simulink model "scenario_2_TAC_5robots_plus_2019"  (R2020a)
settings: Solver=FixedStepAuto  StartTime=0.0  StopTime=60.0  FixedStep=1e-2  RelTol=1e-3
libraries: simulink x5
(part 1 of 2)
settings Model: Creator=Admin  LastModifiedBy=Admin

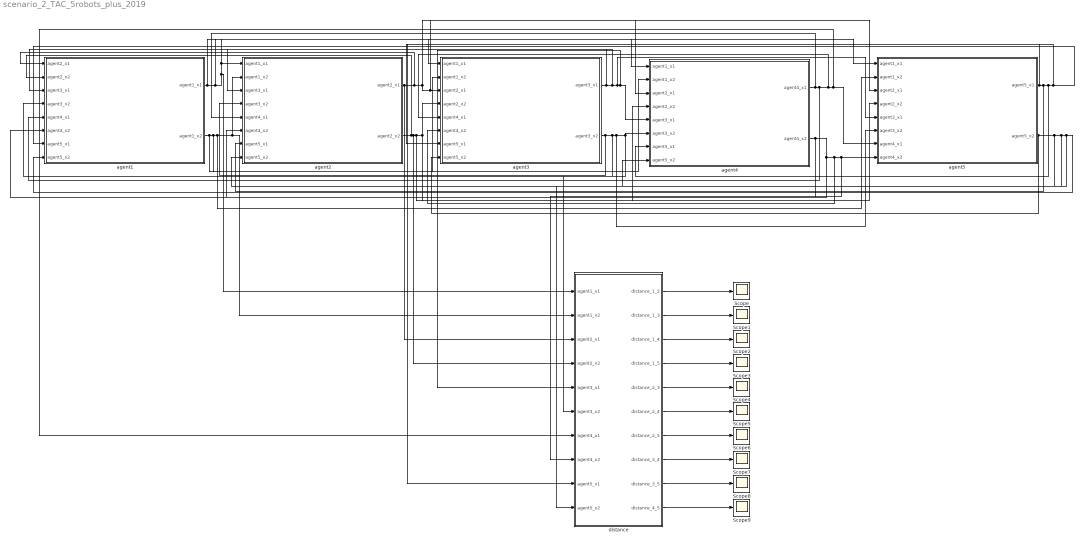
== system scenario_2_TAC_5robots_plus_2019 ==
  Scope{,1..9} (10 alike) : Scope
  agent1 : Subsystem
  agent2 : Subsystem
  agent3 : Subsystem
  agent4 : Subsystem
  agent5 : Subsystem
  distance : MATLAB Function  TreatAsAtomicUnit=on
  wires:
  agent1/1(agent1_x1) -> agent4/1(agent1_x1), agent3/1(agent1_x1), distance/1(agent1_x1), agent5/1(agent1_x1), agent2/1(agent1_x1)
  agent1/2(agent1_x2) -> agent3/2(agent1_x2), agent4/2(agent1_x2), agent5/2(agent1_x2), distance/2(agent1_x2), agent2/2(agent1_x2)
  agent2/1(agent2_x1) -> distance/3(agent2_x1), agent1/1(agent2_x1), agent4/3(agent2_x1), agent3/3(agent2_x1), agent5/3(agent2_x1)
  agent2/2(agent2_x2) -> agent1/2(agent2_x2), distance/4(agent2_x2), agent4/4(agent2_x2), agent5/4(agent2_x2), agent3/4(agent2_x2)
  agent3/1(agent3_x1) -> agent1/3(agent3_x1), agent2/3(agent3_x1), agent5/5(agent3_x1), distance/5(agent3_x1), agent4/5(agent3_x1)
  agent3/2(agent3_x2) -> agent2/4(agent3_x2), agent1/4(agent3_x2), agent5/6(agent3_x2), distance/6(agent3_x2), agent4/6(agent3_x2)
  agent4/1(agent4_x1) -> agent2/5(agent4_x1), agent1/5(agent4_x1), agent3/5(agent4_x1), distance/7(agent4_x1), agent5/7(agent4_x1)
  agent4/2(agent4_x2) -> agent1/6(agent4_x2), agent2/6(agent4_x2), agent3/6(agent4_x2), distance/8(agent4_x2), agent5/8(agent4_x2)
  agent5/1(agent5_x1) -> agent3/7(agent5_x1), agent2/7(agent5_x1), agent4/7(agent5_x1), distance/9(agent5_x1), agent1/7(agent5_x1)
  agent5/2(agent5_x2) -> agent4/8(agent5_x2), distance/10(agent5_x2), agent1/8(agent5_x2), agent2/8(agent5_x2), agent3/8(agent5_x2)
  distance/1(distance_1_2) -> Scope/1
  distance/2(distance_1_3) -> Scope1/1
  distance/3(distance_1_4) -> Scope2/1
  distance/4(distance_1_5) -> Scope3/1
  distance/5(distance_2_3) -> Scope4/1
  distance/6(distance_2_4) -> Scope5/1
  distance/7(distance_2_5) -> Scope6/1
  distance/8(distance_3_4) -> Scope7/1
  distance/9(distance_3_5) -> Scope8/1
  distance/10(distance_4_5) -> Scope9/1

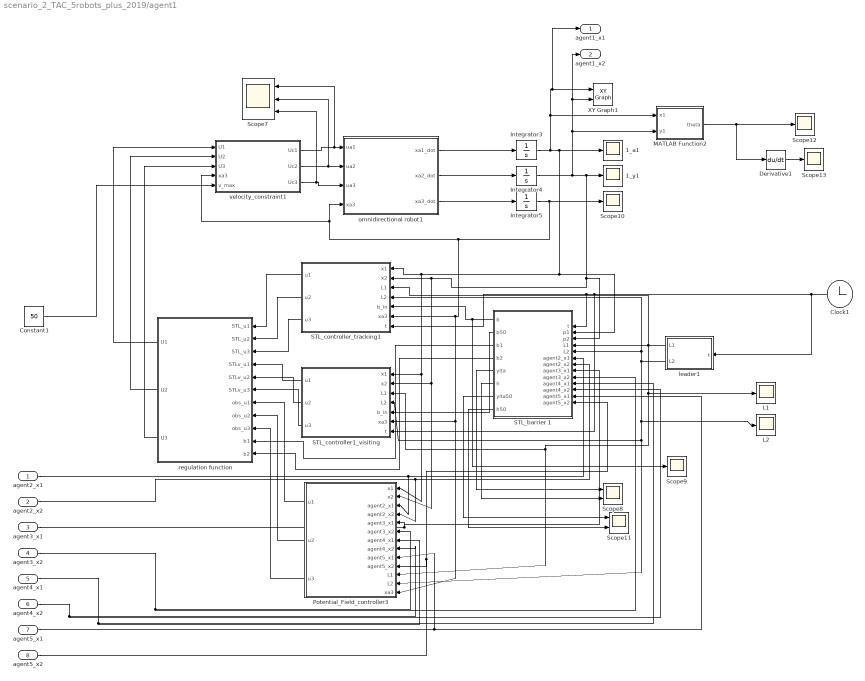
== system scenario_2_TAC_5robots_plus_2019/agent1 ==
  agent2_x1 : Inport
  agent2_x2 : Inport  Port=2
  agent3_x1 : Inport  Port=3
  agent3_x2 : Inport  Port=4
  agent4_x1 : Inport  Port=5
  agent4_x2 : Inport  Port=6
  agent5_x1 : Inport  Port=7
  agent5_x2 : Inport  Port=8
  1_a1 : Scope
  1_y1 : Scope
  Clock1 : Clock
  Constant1 : Constant  Value=50
  Derivative1 : Derivative
  Integrator3 : Integrator
  Integrator4 : Integrator  InitialCondition=10
  Integrator5 : Integrator
  L1 : Scope
  L2 : Scope
  MATLAB Function2 : MATLAB Function  TreatAsAtomicUnit=on
  Potential_Field_controller3 : MATLAB Function  TreatAsAtomicUnit=on
  STL_barrier 1 : MATLAB Function  TreatAsAtomicUnit=on
  STL_controller1_visiting : MATLAB Function  TreatAsAtomicUnit=on
  STL_controller_tracking1 : MATLAB Function  TreatAsAtomicUnit=on
  Scope{9..10,12..13} (4 alike) : Scope
  Scope11 : Scope  NumInputPorts=2
  Scope7 : Scope  NumInputPorts=3
  Scope8 : Scope  NumInputPorts=2
  XY Graph1 : simulink/Sinks/XY Graph  xmin=-60  xmax=60  ymin=-60  ymax=60  st=0.01
  leader1 : MATLAB Function  TreatAsAtomicUnit=on
  omnidirectional robot1 : MATLAB Function  TreatAsAtomicUnit=on
  "regulation function " : MATLAB Function  TreatAsAtomicUnit=on
  velocity_constraint1 : MATLAB Function  TreatAsAtomicUnit=on
  agent1_x1 : Outport
  agent1_x2 : Outport  Port=2
  wires:
  velocity_constraint1/1(Uc1) -> Scope7/1, omnidirectional robot1/1(ua1)
  Integrator3/1 -> MATLAB Function2/1(x1), agent1_x1/1, XY Graph1/1, STL_barrier 1/2(p1), Potential_Field_controller3/1(x1), STL_controller1_visiting/1(x1), STL_controller_tracking1/1(x1), 1_a1/1
  Potential_Field_controller3/3(u3) -> "regulation function "/9(obs_u3)
  omnidirectional robot1/1(xa1_dot) -> Integrator3/1
  leader1/2(L2) -> STL_barrier 1/5(L2), STL_controller_tracking1/4(L2), STL_controller1_visiting/4(L2), Potential_Field_controller3/12(L2), L2/1
  Constant1/1 -> velocity_constraint1/5(v_max)
  STL_barrier 1/4(b2) -> "regulation function "/11(b2)
  Clock1/1 -> STL_controller_tracking1/7(t), STL_barrier 1/1(t), STL_controller1_visiting/7(t), leader1/1(t)
  MATLAB Function2/1(theta) -> Derivative1/1, Scope12/1
  "regulation function "/3(U3) -> velocity_constraint1/3(U3)
  Integrator4/1 -> MATLAB Function2/2(y1), agent1_x2/1, XY Graph1/2, Potential_Field_controller3/2(x2), STL_controller1_visiting/2(x2), STL_controller_tracking1/2(x2), STL_barrier 1/3(p2), 1_y1/1
  omnidirectional robot1/3(xa3_dot) -> Integrator5/1
  STL_controller_tracking1/2(u2) -> "regulation function "/2(STL_u2)
  Potential_Field_controller3/2(u2) -> "regulation function "/8(obs_u2)
  STL_barrier 1/5(yita) -> Scope8/1
  omnidirectional robot1/2(xa2_dot) -> Integrator4/1
  velocity_constraint1/2(Uc2) -> Scope7/2, omnidirectional robot1/2(ua2)
  Potential_Field_controller3/1(u1) -> "regulation function "/7(obs_u1)
  STL_controller_tracking1/3(u3) -> "regulation function "/3(STL_u3)
  STL_barrier 1/6(h) -> Scope8/2
  STL_barrier 1/1(b) -> STL_controller_tracking1/5(b_in), Scope9/1
  STL_barrier 1/3(b1) -> "regulation function "/10(b1)
  STL_barrier 1/8(h50) -> Scope11/2
  velocity_constraint1/3(Uc3) -> Scope7/3, omnidirectional robot1/3(ua3)
  STL_barrier 1/2(b50) -> STL_controller1_visiting/5(b_in)
  "regulation function "/1(U1) -> velocity_constraint1/1(U1)
  leader1/1(L1) -> L1/1, Potential_Field_controller3/11(L1), STL_controller1_visiting/3(L1), STL_barrier 1/4(L1), STL_controller_tracking1/3(L1)
  Integrator5/1 -> velocity_constraint1/4(xa3), omnidirectional robot1/4(xa3), Potential_Field_controller3/13(xa3), STL_controller1_visiting/6(xa3), STL_controller_tracking1/6(xa3), Scope10/1
  Derivative1/1 -> Scope13/1
  STL_barrier 1/7(yita50) -> Scope11/1
  STL_controller1_visiting/3(u3) -> "regulation function "/6(STLv_u3)
  "regulation function "/2(U2) -> velocity_constraint1/2(U2)
  STL_controller1_visiting/1(u1) -> "regulation function "/4(STLv_u1)
  STL_controller1_visiting/2(u2) -> "regulation function "/5(STLv_u2)
  STL_controller_tracking1/1(u1) -> "regulation function "/1(STL_u1)
  agent2_x1/1 -> STL_barrier 1/6(agent2_x1), Potential_Field_controller3/3(agent2_x1)
  agent2_x2/1 -> STL_barrier 1/7(agent2_x2), Potential_Field_controller3/4(agent2_x2)
  agent3_x1/1 -> STL_barrier 1/8(agent3_x1), Potential_Field_controller3/5(agent3_x1)
  agent3_x2/1 -> STL_barrier 1/9(agent3_x2), Potential_Field_controller3/6(agent3_x2)
  agent4_x1/1 -> STL_barrier 1/10(agent4_x1), Potential_Field_controller3/7(agent4_x1)
  agent4_x2/1 -> STL_barrier 1/11(agent4_x2), Potential_Field_controller3/8(agent4_x2)
  agent5_x1/1 -> STL_barrier 1/12(agent5_x1), Potential_Field_controller3/9(agent5_x1)
  agent5_x2/1 -> STL_barrier 1/13(agent5_x2), Potential_Field_controller3/10(agent5_x2)

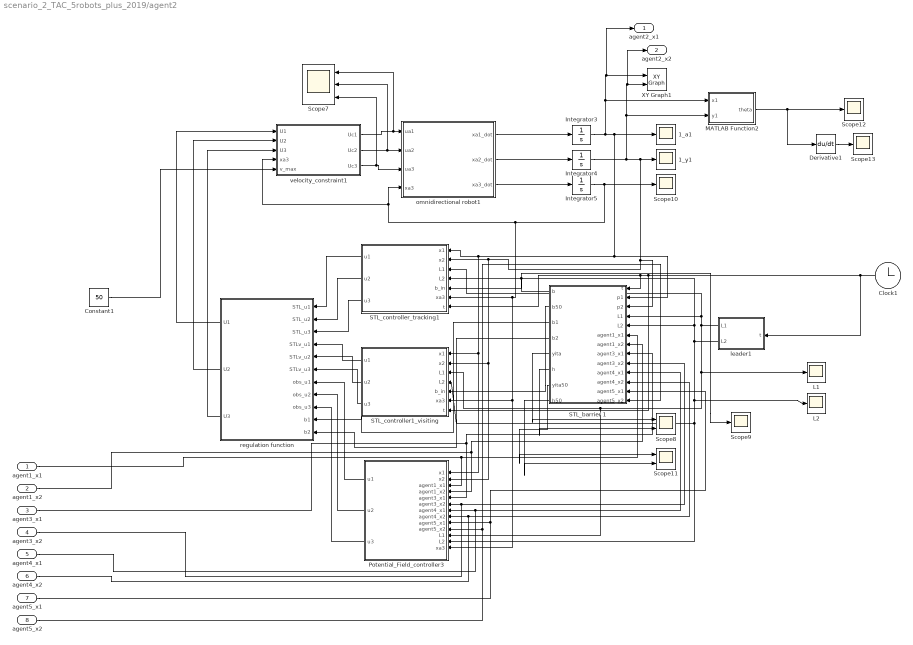
== system scenario_2_TAC_5robots_plus_2019/agent2 ==
  agent1_x1 : Inport
  agent1_x2 : Inport  Port=2
  agent3_x1 : Inport  Port=3
  agent3_x2 : Inport  Port=4
  agent4_x1 : Inport  Port=5
  agent4_x2 : Inport  Port=6
  agent5_x1 : Inport  Port=7
  agent5_x2 : Inport  Port=8
  1_a1 : Scope
  1_y1 : Scope
  Clock1 : Clock
  Constant1 : Constant  Value=50
  Derivative1 : Derivative
  Integrator3 : Integrator  InitialCondition=10
  Integrator4 : Integrator
  Integrator5 : Integrator
  L1 : Scope
  L2 : Scope
  MATLAB Function2 : MATLAB Function  TreatAsAtomicUnit=on
  Potential_Field_controller3 : MATLAB Function  TreatAsAtomicUnit=on
  STL_barrier 1 : MATLAB Function  TreatAsAtomicUnit=on
  STL_controller1_visiting : MATLAB Function  TreatAsAtomicUnit=on
  STL_controller_tracking1 : MATLAB Function  TreatAsAtomicUnit=on
  Scope{9..10,12..13} (4 alike) : Scope
  Scope11 : Scope  NumInputPorts=2
  Scope7 : Scope  NumInputPorts=3
  Scope8 : Scope  NumInputPorts=2
  XY Graph1 : simulink/Sinks/XY Graph  xmin=-60  xmax=60  ymin=-60  ymax=60  st=0.01
  leader1 : MATLAB Function  TreatAsAtomicUnit=on
  omnidirectional robot1 : MATLAB Function  TreatAsAtomicUnit=on
  "regulation function " : MATLAB Function  TreatAsAtomicUnit=on
  velocity_constraint1 : MATLAB Function  TreatAsAtomicUnit=on
  agent2_x1 : Outport
  agent2_x2 : Outport  Port=2
  wires:
  velocity_constraint1/1(Uc1) -> Scope7/1, omnidirectional robot1/1(ua1)
  Integrator3/1 -> MATLAB Function2/1(x1), agent2_x1/1, XY Graph1/1, STL_barrier 1/2(p1), Potential_Field_controller3/1(x1), STL_controller1_visiting/1(x1), STL_controller_tracking1/1(x1), 1_a1/1
  Potential_Field_controller3/3(u3) -> "regulation function "/9(obs_u3)
  omnidirectional robot1/1(xa1_dot) -> Integrator3/1
  leader1/2(L2) -> STL_controller_tracking1/4(L2), STL_barrier 1/5(L2), STL_controller1_visiting/4(L2), Potential_Field_controller3/12(L2), L2/1
  Constant1/1 -> velocity_constraint1/5(v_max)
  STL_barrier 1/4(b2) -> "regulation function "/11(b2)
  Clock1/1 -> STL_controller_tracking1/7(t), STL_barrier 1/1(t), STL_controller1_visiting/7(t), leader1/1(t)
  MATLAB Function2/1(theta) -> Derivative1/1, Scope12/1
  "regulation function "/3(U3) -> velocity_constraint1/3(U3)
  Integrator4/1 -> MATLAB Function2/2(y1), agent2_x2/1, XY Graph1/2, Potential_Field_controller3/2(x2), STL_controller1_visiting/2(x2), STL_controller_tracking1/2(x2), STL_barrier 1/3(p2), 1_y1/1
  omnidirectional robot1/3(xa3_dot) -> Integrator5/1
  STL_controller_tracking1/2(u2) -> "regulation function "/2(STL_u2)
  Potential_Field_controller3/2(u2) -> "regulation function "/8(obs_u2)
  STL_barrier 1/5(yita) -> Scope8/1
  omnidirectional robot1/2(xa2_dot) -> Integrator4/1
  velocity_constraint1/2(Uc2) -> Scope7/2, omnidirectional robot1/2(ua2)
  Potential_Field_controller3/1(u1) -> "regulation function "/7(obs_u1)
  STL_controller_tracking1/3(u3) -> "regulation function "/3(STL_u3)
  STL_barrier 1/6(h) -> Scope8/2
  STL_barrier 1/1(b) -> STL_controller_tracking1/5(b_in), Scope9/1
  STL_barrier 1/3(b1) -> "regulation function "/10(b1)
  STL_barrier 1/8(h50) -> Scope11/2
  velocity_constraint1/3(Uc3) -> Scope7/3, omnidirectional robot1/3(ua3)
  STL_barrier 1/2(b50) -> STL_controller1_visiting/5(b_in)
  "regulation function "/1(U1) -> velocity_constraint1/1(U1)
  leader1/1(L1) -> STL_controller_tracking1/3(L1), STL_barrier 1/4(L1), L1/1, STL_controller1_visiting/3(L1), Potential_Field_controller3/11(L1)
  Integrator5/1 -> velocity_constraint1/4(xa3), omnidirectional robot1/4(xa3), Potential_Field_controller3/13(xa3), STL_controller1_visiting/6(xa3), STL_controller_tracking1/6(xa3), Scope10/1
  Derivative1/1 -> Scope13/1
  STL_barrier 1/7(yita50) -> Scope11/1
  STL_controller1_visiting/3(u3) -> "regulation function "/6(STLv_u3)
  "regulation function "/2(U2) -> velocity_constraint1/2(U2)
  STL_controller1_visiting/1(u1) -> "regulation function "/4(STLv_u1)
  STL_controller1_visiting/2(u2) -> "regulation function "/5(STLv_u2)
  STL_controller_tracking1/1(u1) -> "regulation function "/1(STL_u1)
  agent1_x1/1 -> STL_barrier 1/6(agent1_x1), Potential_Field_controller3/3(agent1_x1)
  agent1_x2/1 -> STL_barrier 1/7(agent1_x2), Potential_Field_controller3/4(agent1_x2)
  agent3_x1/1 -> STL_barrier 1/8(agent3_x1), Potential_Field_controller3/5(agent3_x1)
  agent3_x2/1 -> STL_barrier 1/9(agent3_x2), Potential_Field_controller3/6(agent3_x2)
  agent4_x1/1 -> STL_barrier 1/10(agent4_x1), Potential_Field_controller3/7(agent4_x1)
  agent4_x2/1 -> STL_barrier 1/11(agent4_x2), Potential_Field_controller3/8(agent4_x2)
  agent5_x1/1 -> STL_barrier 1/12(agent5_x1), Potential_Field_controller3/9(agent5_x1)
  agent5_x2/1 -> STL_barrier 1/13(agent5_x2), Potential_Field_controller3/10(agent5_x2)

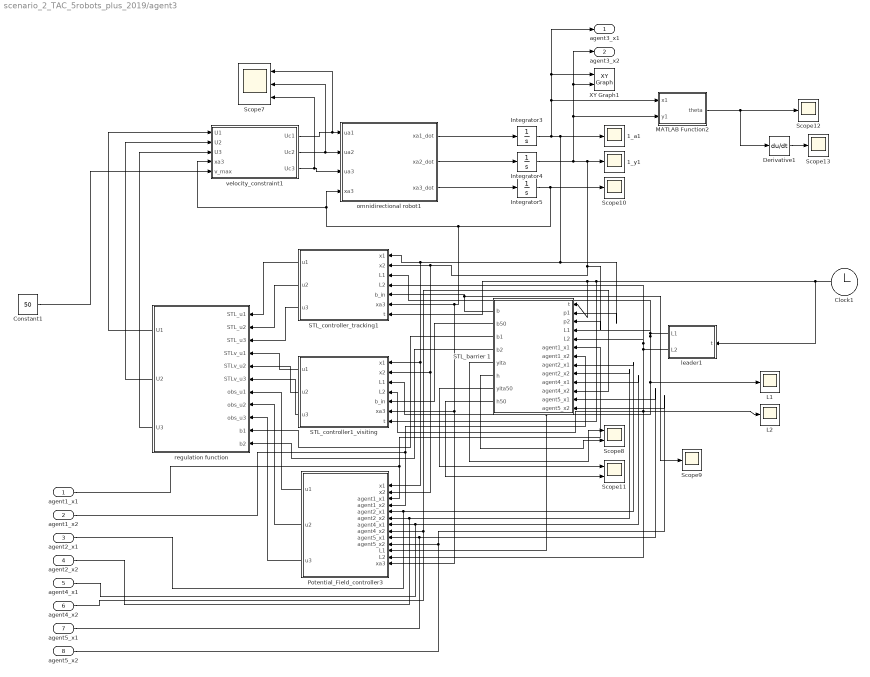
== system scenario_2_TAC_5robots_plus_2019/agent3 ==
  agent1_x1 : Inport
  agent1_x2 : Inport  Port=2
  agent2_x1 : Inport  Port=3
  agent2_x2 : Inport  Port=4
  agent4_x1 : Inport  Port=5
  agent4_x2 : Inport  Port=6
  agent5_x1 : Inport  Port=7
  agent5_x2 : Inport  Port=8
  1_a1 : Scope
  1_y1 : Scope
  Clock1 : Clock
  Constant1 : Constant  Value=50
  Derivative1 : Derivative
  Integrator3 : Integrator
  Integrator4 : Integrator  InitialCondition=-10
  Integrator5 : Integrator
  L1 : Scope
  L2 : Scope
  MATLAB Function2 : MATLAB Function  TreatAsAtomicUnit=on
  Potential_Field_controller3 : MATLAB Function  TreatAsAtomicUnit=on
  STL_barrier 1 : MATLAB Function  TreatAsAtomicUnit=on
  STL_controller1_visiting : MATLAB Function  TreatAsAtomicUnit=on
  STL_controller_tracking1 : MATLAB Function  TreatAsAtomicUnit=on
  Scope{9..10,12..13} (4 alike) : Scope
  Scope11 : Scope  NumInputPorts=2
  Scope7 : Scope  NumInputPorts=3
  Scope8 : Scope  NumInputPorts=2
  XY Graph1 : simulink/Sinks/XY Graph  xmin=-60  xmax=60  ymin=-60  ymax=60  st=0.01
  leader1 : MATLAB Function  TreatAsAtomicUnit=on
  omnidirectional robot1 : MATLAB Function  TreatAsAtomicUnit=on
  "regulation function " : MATLAB Function  TreatAsAtomicUnit=on
  velocity_constraint1 : MATLAB Function  TreatAsAtomicUnit=on
  agent3_x1 : Outport
  agent3_x2 : Outport  Port=2
  wires:
  velocity_constraint1/1(Uc1) -> Scope7/1, omnidirectional robot1/1(ua1)
  Integrator3/1 -> MATLAB Function2/1(x1), agent3_x1/1, XY Graph1/1, STL_barrier 1/2(p1), Potential_Field_controller3/1(x1), STL_controller1_visiting/1(x1), STL_controller_tracking1/1(x1), 1_a1/1
  Potential_Field_controller3/3(u3) -> "regulation function "/9(obs_u3)
  omnidirectional robot1/1(xa1_dot) -> Integrator3/1
  leader1/2(L2) -> STL_controller_tracking1/4(L2), STL_barrier 1/5(L2), STL_controller1_visiting/4(L2), Potential_Field_controller3/12(L2), L2/1
  Constant1/1 -> velocity_constraint1/5(v_max)
  STL_barrier 1/4(b2) -> "regulation function "/11(b2)
  Clock1/1 -> STL_controller_tracking1/7(t), STL_barrier 1/1(t), STL_controller1_visiting/7(t), leader1/1(t)
  MATLAB Function2/1(theta) -> Derivative1/1, Scope12/1
  "regulation function "/3(U3) -> velocity_constraint1/3(U3)
  Integrator4/1 -> MATLAB Function2/2(y1), XY Graph1/2, agent3_x2/1, Potential_Field_controller3/2(x2), STL_controller1_visiting/2(x2), STL_controller_tracking1/2(x2), STL_barrier 1/3(p2), 1_y1/1
  omnidirectional robot1/3(xa3_dot) -> Integrator5/1
  STL_controller_tracking1/2(u2) -> "regulation function "/2(STL_u2)
  Potential_Field_controller3/2(u2) -> "regulation function "/8(obs_u2)
  STL_barrier 1/5(yita) -> Scope8/1
  omnidirectional robot1/2(xa2_dot) -> Integrator4/1
  velocity_constraint1/2(Uc2) -> Scope7/2, omnidirectional robot1/2(ua2)
  Potential_Field_controller3/1(u1) -> "regulation function "/7(obs_u1)
  STL_controller_tracking1/3(u3) -> "regulation function "/3(STL_u3)
  STL_barrier 1/6(h) -> Scope8/2
  STL_barrier 1/1(b) -> STL_controller_tracking1/5(b_in), Scope9/1
  STL_barrier 1/3(b1) -> "regulation function "/10(b1)
  STL_barrier 1/8(h50) -> Scope11/2
  velocity_constraint1/3(Uc3) -> Scope7/3, omnidirectional robot1/3(ua3)
  STL_barrier 1/2(b50) -> STL_controller1_visiting/5(b_in)
  "regulation function "/1(U1) -> velocity_constraint1/1(U1)
  leader1/1(L1) -> STL_barrier 1/4(L1), L1/1, STL_controller1_visiting/3(L1), Potential_Field_controller3/11(L1), STL_controller_tracking1/3(L1)
  Integrator5/1 -> velocity_constraint1/4(xa3), omnidirectional robot1/4(xa3), Potential_Field_controller3/13(xa3), STL_controller1_visiting/6(xa3), STL_controller_tracking1/6(xa3), Scope10/1
  Derivative1/1 -> Scope13/1
  STL_barrier 1/7(yita50) -> Scope11/1
  STL_controller1_visiting/3(u3) -> "regulation function "/6(STLv_u3)
  "regulation function "/2(U2) -> velocity_constraint1/2(U2)
  STL_controller1_visiting/1(u1) -> "regulation function "/4(STLv_u1)
  STL_controller1_visiting/2(u2) -> "regulation function "/5(STLv_u2)
  STL_controller_tracking1/1(u1) -> "regulation function "/1(STL_u1)
  agent1_x1/1 -> STL_barrier 1/6(agent1_x1), Potential_Field_controller3/3(agent1_x1)
  agent1_x2/1 -> STL_barrier 1/7(agent1_x2), Potential_Field_controller3/4(agent1_x2)
  agent2_x1/1 -> STL_barrier 1/8(agent2_x1), Potential_Field_controller3/5(agent2_x1)
  agent2_x2/1 -> STL_barrier 1/9(agent2_x2), Potential_Field_controller3/6(agent2_x2)
  agent4_x1/1 -> STL_barrier 1/10(agent4_x1), Potential_Field_controller3/7(agent4_x1)
  agent4_x2/1 -> STL_barrier 1/11(agent4_x2), Potential_Field_controller3/8(agent4_x2)
  agent5_x1/1 -> STL_barrier 1/12(agent5_x1), Potential_Field_controller3/9(agent5_x1)
  agent5_x2/1 -> STL_barrier 1/13(agent5_x2), Potential_Field_controller3/10(agent5_x2)

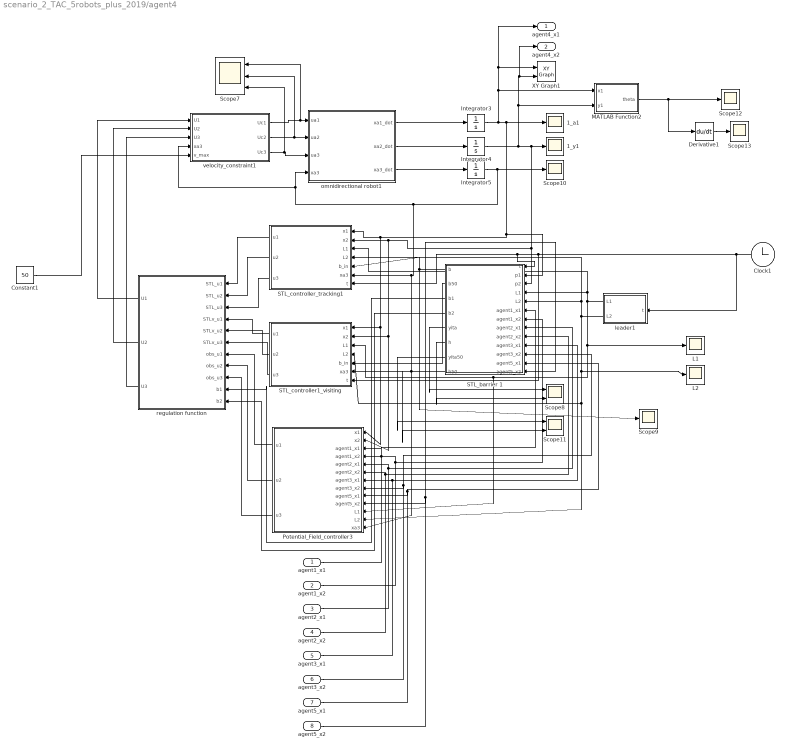
== system scenario_2_TAC_5robots_plus_2019/agent4 ==
  agent1_x1 : Inport
  agent1_x2 : Inport  Port=2
  agent2_x1 : Inport  Port=3
  agent2_x2 : Inport  Port=4
  agent3_x1 : Inport  Port=5
  agent3_x2 : Inport  Port=6
  agent5_x1 : Inport  Port=7
  agent5_x2 : Inport  Port=8
  1_a1 : Scope
  1_y1 : Scope
  Clock1 : Clock
  Constant1 : Constant  Value=50
  Derivative1 : Derivative
  Integrator3 : Integrator  InitialCondition=-10
  Integrator4 : Integrator
  Integrator5 : Integrator
  L1 : Scope
  L2 : Scope
  MATLAB Function2 : MATLAB Function  TreatAsAtomicUnit=on
  Potential_Field_controller3 : MATLAB Function  TreatAsAtomicUnit=on
  STL_barrier 1 : MATLAB Function  TreatAsAtomicUnit=on
  STL_controller1_visiting : MATLAB Function  TreatAsAtomicUnit=on
  STL_controller_tracking1 : MATLAB Function  TreatAsAtomicUnit=on
  Scope{9..10,12..13} (4 alike) : Scope
  Scope11 : Scope  NumInputPorts=2
  Scope7 : Scope  NumInputPorts=3
  Scope8 : Scope  NumInputPorts=2
  XY Graph1 : simulink/Sinks/XY Graph  xmin=-60  xmax=60  ymin=-60  ymax=60  st=0.01
  leader1 : MATLAB Function  TreatAsAtomicUnit=on
  omnidirectional robot1 : MATLAB Function  TreatAsAtomicUnit=on
  "regulation function " : MATLAB Function  TreatAsAtomicUnit=on
  velocity_constraint1 : MATLAB Function  TreatAsAtomicUnit=on
  agent4_x1 : Outport
  agent4_x2 : Outport  Port=2
  wires:
  velocity_constraint1/1(Uc1) -> Scope7/1, omnidirectional robot1/1(ua1)
  Integrator3/1 -> MATLAB Function2/1(x1), agent4_x1/1, XY Graph1/1, Potential_Field_controller3/1(x1), STL_controller1_visiting/1(x1), STL_controller_tracking1/1(x1), STL_barrier 1/2(p1), 1_a1/1
  Potential_Field_controller3/3(u3) -> "regulation function "/9(obs_u3)
  omnidirectional robot1/1(xa1_dot) -> Integrator3/1
  leader1/2(L2) -> STL_controller_tracking1/4(L2), STL_barrier 1/5(L2), STL_controller1_visiting/4(L2), Potential_Field_controller3/12(L2), L2/1
  Constant1/1 -> velocity_constraint1/5(v_max)
  STL_barrier 1/4(b2) -> "regulation function "/11(b2)
  Clock1/1 -> STL_barrier 1/1(t), STL_controller_tracking1/7(t), STL_controller1_visiting/7(t), leader1/1(t)
  MATLAB Function2/1(theta) -> Derivative1/1, Scope12/1
  "regulation function "/3(U3) -> velocity_constraint1/3(U3)
  Integrator4/1 -> MATLAB Function2/2(y1), agent4_x2/1, XY Graph1/2, STL_barrier 1/3(p2), Potential_Field_controller3/2(x2), STL_controller1_visiting/2(x2), STL_controller_tracking1/2(x2), 1_y1/1
  omnidirectional robot1/3(xa3_dot) -> Integrator5/1
  STL_controller_tracking1/2(u2) -> "regulation function "/2(STL_u2)
  Potential_Field_controller3/2(u2) -> "regulation function "/8(obs_u2)
  STL_barrier 1/5(yita) -> Scope8/1
  omnidirectional robot1/2(xa2_dot) -> Integrator4/1
  velocity_constraint1/2(Uc2) -> Scope7/2, omnidirectional robot1/2(ua2)
  Potential_Field_controller3/1(u1) -> "regulation function "/7(obs_u1)
  STL_controller_tracking1/3(u3) -> "regulation function "/3(STL_u3)
  STL_barrier 1/6(h) -> Scope8/2
  STL_barrier 1/1(b) -> STL_controller_tracking1/5(b_in), Scope9/1
  STL_barrier 1/3(b1) -> "regulation function "/10(b1)
  STL_barrier 1/8(h50) -> Scope11/2
  velocity_constraint1/3(Uc3) -> Scope7/3, omnidirectional robot1/3(ua3)
  STL_barrier 1/2(b50) -> STL_controller1_visiting/5(b_in)
  "regulation function "/1(U1) -> velocity_constraint1/1(U1)
  leader1/1(L1) -> STL_controller_tracking1/3(L1), STL_barrier 1/4(L1), L1/1, Potential_Field_controller3/11(L1), STL_controller1_visiting/3(L1)
  Integrator5/1 -> velocity_constraint1/4(xa3), omnidirectional robot1/4(xa3), Potential_Field_controller3/13(xa3), STL_controller1_visiting/6(xa3), STL_controller_tracking1/6(xa3), Scope10/1
  Derivative1/1 -> Scope13/1
  STL_barrier 1/7(yita50) -> Scope11/1
  STL_controller1_visiting/3(u3) -> "regulation function "/6(STLv_u3)
  "regulation function "/2(U2) -> velocity_constraint1/2(U2)
  STL_controller1_visiting/1(u1) -> "regulation function "/4(STLv_u1)
  STL_controller1_visiting/2(u2) -> "regulation function "/5(STLv_u2)
  STL_controller_tracking1/1(u1) -> "regulation function "/1(STL_u1)
  agent1_x1/1 -> STL_barrier 1/6(agent1_x1), Potential_Field_controller3/3(agent1_x1)
  agent1_x2/1 -> STL_barrier 1/7(agent1_x2), Potential_Field_controller3/4(agent1_x2)
  agent2_x1/1 -> STL_barrier 1/8(agent2_x1), Potential_Field_controller3/5(agent2_x1)
  agent2_x2/1 -> STL_barrier 1/9(agent2_x2), Potential_Field_controller3/6(agent2_x2)
  agent3_x1/1 -> STL_barrier 1/10(agent3_x1), Potential_Field_controller3/7(agent3_x1)
  agent3_x2/1 -> STL_barrier 1/11(agent3_x2), Potential_Field_controller3/8(agent3_x2)
  agent5_x1/1 -> STL_barrier 1/12(agent5_x1), Potential_Field_controller3/9(agent5_x1)
  agent5_x2/1 -> STL_barrier 1/13(agent5_x2), Potential_Field_controller3/10(agent5_x2)

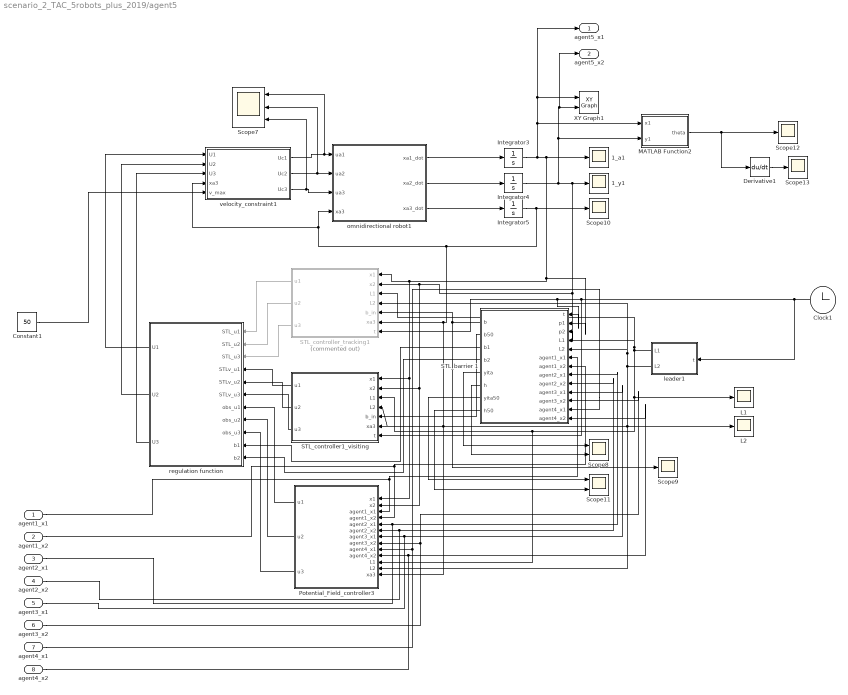
== system scenario_2_TAC_5robots_plus_2019/agent5 ==
  agent1_x1 : Inport
  agent1_x2 : Inport  Port=2
  agent2_x1 : Inport  Port=3
  agent2_x2 : Inport  Port=4
  agent3_x1 : Inport  Port=5
  agent3_x2 : Inport  Port=6
  agent4_x1 : Inport  Port=7
  agent4_x2 : Inport  Port=8
  1_a1 : Scope
  1_y1 : Scope
  Clock1 : Clock
  Constant1 : Constant  Value=50
  Derivative1 : Derivative
  Integrator3 : Integrator  InitialCondition=-60
  Integrator4 : Integrator
  Integrator5 : Integrator
  L1 : Scope
  L2 : Scope
  MATLAB Function2 : MATLAB Function  TreatAsAtomicUnit=on
  Potential_Field_controller3 : MATLAB Function  TreatAsAtomicUnit=on
  STL_barrier 1 : MATLAB Function  TreatAsAtomicUnit=on
  STL_controller1_visiting : MATLAB Function  TreatAsAtomicUnit=on
  STL_controller_tracking1 : MATLAB Function  Commented=on  TreatAsAtomicUnit=on
  Scope{9..10,12..13} (4 alike) : Scope
  Scope11 : Scope  NumInputPorts=2
  Scope7 : Scope  NumInputPorts=3
  Scope8 : Scope  NumInputPorts=2
  XY Graph1 : simulink/Sinks/XY Graph  xmin=-60  xmax=60  ymin=-60  ymax=60  st=0.01
  leader1 : MATLAB Function  TreatAsAtomicUnit=on
  omnidirectional robot1 : MATLAB Function  TreatAsAtomicUnit=on
  "regulation function " : MATLAB Function  TreatAsAtomicUnit=on
  velocity_constraint1 : MATLAB Function  TreatAsAtomicUnit=on
  agent5_x1 : Outport
  agent5_x2 : Outport  Port=2
  wires:
  velocity_constraint1/1(Uc1) -> Scope7/1, omnidirectional robot1/1(ua1)
  Integrator3/1 -> MATLAB Function2/1(x1), agent5_x1/1, XY Graph1/1, Potential_Field_controller3/1(x1), STL_controller1_visiting/1(x1), STL_controller_tracking1/1(x1), STL_barrier 1/2(p1), 1_a1/1
  Potential_Field_controller3/3(u3) -> "regulation function "/9(obs_u3)
  omnidirectional robot1/1(xa1_dot) -> Integrator3/1
  leader1/2(L2) -> STL_controller_tracking1/4(L2), STL_barrier 1/5(L2), STL_controller1_visiting/4(L2), Potential_Field_controller3/12(L2), L2/1
  Constant1/1 -> velocity_constraint1/5(v_max)
  STL_barrier 1/4(b2) -> "regulation function "/11(b2)
  Clock1/1 -> STL_barrier 1/1(t), STL_controller_tracking1/7(t), STL_controller1_visiting/7(t), leader1/1(t)
  MATLAB Function2/1(theta) -> Derivative1/1, Scope12/1
  "regulation function "/3(U3) -> velocity_constraint1/3(U3)
  Integrator4/1 -> MATLAB Function2/2(y1), agent5_x2/1, XY Graph1/2, STL_barrier 1/3(p2), Potential_Field_controller3/2(x2), STL_controller1_visiting/2(x2), STL_controller_tracking1/2(x2), 1_y1/1
  omnidirectional robot1/3(xa3_dot) -> Integrator5/1
  STL_controller_tracking1/2(u2) -> "regulation function "/2(STL_u2)
  Potential_Field_controller3/2(u2) -> "regulation function "/8(obs_u2)
  STL_barrier 1/5(yita) -> Scope8/1
  omnidirectional robot1/2(xa2_dot) -> Integrator4/1
  velocity_constraint1/2(Uc2) -> Scope7/2, omnidirectional robot1/2(ua2)
  Potential_Field_controller3/1(u1) -> "regulation function "/7(obs_u1)
  STL_controller_tracking1/3(u3) -> "regulation function "/3(STL_u3)
  STL_barrier 1/6(h) -> Scope8/2
  STL_barrier 1/1(b) -> STL_controller_tracking1/5(b_in), Scope9/1
  STL_barrier 1/3(b1) -> "regulation function "/10(b1)
  STL_barrier 1/8(h50) -> Scope11/2
  velocity_constraint1/3(Uc3) -> Scope7/3, omnidirectional robot1/3(ua3)
  STL_barrier 1/2(b50) -> STL_controller1_visiting/5(b_in)
  "regulation function "/1(U1) -> velocity_constraint1/1(U1)
  leader1/1(L1) -> STL_controller_tracking1/3(L1), STL_barrier 1/4(L1), L1/1, STL_controller1_visiting/3(L1), Potential_Field_controller3/11(L1)
  Integrator5/1 -> velocity_constraint1/4(xa3), omnidirectional robot1/4(xa3), Potential_Field_controller3/13(xa3), STL_controller1_visiting/6(xa3), STL_controller_tracking1/6(xa3), Scope10/1
  Derivative1/1 -> Scope13/1
  STL_barrier 1/7(yita50) -> Scope11/1
  STL_controller1_visiting/3(u3) -> "regulation function "/6(STLv_u3)
  "regulation function "/2(U2) -> velocity_constraint1/2(U2)
  STL_controller1_visiting/1(u1) -> "regulation function "/4(STLv_u1)
  STL_controller1_visiting/2(u2) -> "regulation function "/5(STLv_u2)
  STL_controller_tracking1/1(u1) -> "regulation function "/1(STL_u1)
  agent1_x1/1 -> STL_barrier 1/6(agent1_x1), Potential_Field_controller3/3(agent1_x1)
  agent1_x2/1 -> STL_barrier 1/7(agent1_x2), Potential_Field_controller3/4(agent1_x2)
  agent2_x1/1 -> STL_barrier 1/8(agent2_x1), Potential_Field_controller3/5(agent2_x1)
  agent2_x2/1 -> STL_barrier 1/9(agent2_x2), Potential_Field_controller3/6(agent2_x2)
  agent3_x1/1 -> STL_barrier 1/10(agent3_x1), Potential_Field_controller3/7(agent3_x1)
  agent3_x2/1 -> STL_barrier 1/11(agent3_x2), Potential_Field_controller3/8(agent3_x2)
  agent4_x1/1 -> STL_barrier 1/12(agent4_x1), Potential_Field_controller3/9(agent4_x1)
  agent4_x2/1 -> STL_barrier 1/13(agent4_x2), Potential_Field_controller3/10(agent4_x2)

== matlab function scenario_2_TAC_5robots_plus_2019/agent2/STL_controller_tracking1 ==
  data: x1 input; x2 input; L1 input; L2 input; b_in input; u1 output; xa3 input; u2 output; u3 output; t input
function [u1,u2,u3]= fcn(x1, x2,L1,L2, b_in, xa3,t)
coder.extrinsic('quadoptimizer');
%coder.extrinsic('save');
d1=L1; d2=L2;

partial_b=(1/2)*((x1-d1)^2+(x2-d2)^2)^(-1/2);
partial_b_x=[-2*partial_b*(x1-d1),-2*partial_b*(x2-d2),0];
partial_b_L=[2*partial_b*(x1-d1),2*partial_b*(x2-d2)];
pho1=sqrt(partial_b_L(1,1)^2+partial_b_L(1,2)^2);
Li=0.2;
Bi=[0,cos(pi/6),-cos(pi/6);
    -1,sin(pi/6),sin(pi/6);
    Li,Li,Li;];

R1=[cos(xa3),-sin(xa3),0;
    sin(xa3),cos(xa3),0;
    0,0,1;];
R=0.02;

gx=R1*inv(Bi')*R;

A=partial_b_x*gx;

H=[1,0,0;0,1,0;0,0,1];
%H=[1];

% b=200*b_in-0.37*25*exp(-0.37*t)-300-30*pho1;
b=200*b_in-0.32*25*exp(-0.32*t)-300-30*pho1;


u1=0;u2=0;u3=0;
U=quadoptimizer(H,b,A);

%U=quadprod(H,[],-A,b);

u1=U(1,1);
u2=U(2,1);
u3=U(3,1);

== matlab function scenario_2_TAC_5robots_plus_2019/agent2/leader1 ==
  data: t input; L1 output; L2 output
function [L1,L2] = fcn(t)
L1=30*cos(1*t);
L2=-30*sin(1*t);

== matlab function scenario_2_TAC_5robots_plus_2019/agent2/omnidirectional robot1 ==
  data: ua1 input; xa1_dot output; ua2 input; ua3 input; xa3 input; xa2_dot output; xa3_dot output
function [xa1_dot,xa2_dot,xa3_dot]= fcn(ua1,ua2,ua3,xa3)

Li=0.2;
Bi=[0,cos(pi/6),-cos(pi/6);
    -1,sin(pi/6),sin(pi/6);
    Li,Li,Li;];

R1=[cos(xa3),-sin(xa3),0;
    sin(xa3),cos(xa3),0;
    0,0,1;];
R=0.02;

A=R1*inv(Bi')*R*[ua1;ua2;ua3];
xa1_dot=A(1,1);
xa2_dot=A(2,1);
xa3_dot=A(3,1);

== matlab function scenario_2_TAC_5robots_plus_2019/agent2/regulation function  ==
  data: STL_u1 input; U1 output; STL_u2 input; STL_u3 input; STLv_u1 input; STLv_u2 input; STLv_u3 input; obs_u1 input; obs_u2 input; obs_u3 input; b1 input; U2 output; U3 output; b2 input
function [U1,U2,U3] = fcn(STL_u1,STL_u2,STL_u3,STLv_u1,STLv_u2,STLv_u3,obs_u1,obs_u2,obs_u3,b1,b2)
U_track=[STL_u1;STL_u2;STL_u3];
U_visit=[STLv_u1;STLv_u2;STLv_u3];
U_obs=[obs_u1;obs_u2;obs_u3];

k=0.065;
lambda=1-exp(-k*max(b1,0));
U_goal=lambda*U_track+(1-lambda)*U_visit;
% U_goal=[0;0;0];
% U_goal=U_track;
j=0.15;
gamma=1-exp(-j*max(b2,0));
U=gamma*U_goal+(1-gamma)*U_obs;

% U=U_goal;
U1=0;U2=0;U3=0;
U1=U(1,1);
U2=U(2,1);
U3=U(3,1);

== matlab function scenario_2_TAC_5robots_plus_2019/agent2/velocity_constraint1 ==
  data: U1 input; Uc1 output; U2 input; U3 input; xa3 input; v_max input; Uc2 output; Uc3 output
function [Uc1,Uc2,Uc3] = fcn(U1,U2,U3,xa3,v_max)

Li=0.2;
Bi=[0,cos(pi/6),-cos(pi/6);
    -1,sin(pi/6),sin(pi/6);
    Li,Li,Li;];

R1=[cos(xa3),-sin(xa3),0;
    sin(xa3),cos(xa3),0;
    0,0,1;];
R=0.02;
gx=R1*inv(Bi')*R;

U=[U1;U2;U3];
V=[0;0;0];
V=gx*U;
if V(1,1)^2+V(2,1)^2<=v_max^2
     U(1,1)= U(1,1);
     U(2,1)= U(2,1);
else 
    U(1,1)=sqrt(v_max^2/(V(1,1)^2+V(2,1)^2))*U(1,1);
    U(2,1)=sqrt(v_max^2/(V(1,1)^2+V(2,1)^2))*U(2,1);
    U(3,1)=sqrt(v_max^2/(V(1,1)^2+V(2,1)^2))*U(3,1);
end

Uc1=U(1,1);
Uc2=U(2,1);
Uc3=U(3,1);

== matlab function scenario_2_TAC_5robots_plus_2019/agent3/MATLAB Function2 ==
  data: x1 input; theta output; y1 input
function theta = fcn(x1, y1)
theta=atan2(y1,x1);

== matlab function scenario_2_TAC_5robots_plus_2019/agent3/Potential_Field_controller3 ==
  data: x1 input; x2 input; agent1_x1 input; agent1_x2 input; agent2_x1 input; agent2_x2 input; agent4_x1 input; agent4_x2 input; agent5_x1 input; agent5_x2 input; L1 input; L2 input; u1 output; xa3 input; u2 output; u3 output
function [u1,u2,u3] = fcn(x1, x2,agent1_x1,agent1_x2,agent2_x1,agent2_x2,agent4_x1,agent4_x2,agent5_x1,agent5_x2,L1,L2, xa3)
coder.extrinsic('Calculate_gradient');
coder.extrinsic('Calculate_gradient_x15');
coder.extrinsic('PVF_optimizer');
coder.extrinsic('add_random');
A1=[-1,0;0,-1];
F=[2*L1,2*L2];
distance=sqrt((x1-90)^2+(x2-90)^2);

gradient_x=0;gradient_y=0;
agent1_gradient_x=0;agent1_gradient_y=0;
agent2_gradient_x=0;agent2_gradient_y=0;
agent4_gradient_x=0;agent4_gradient_y=0;
agent5_gradient_x=0;agent5_gradient_y=0;
[gradient_x,gradient_y]=Calculate_gradient(x1,x2,A1,F,0,30,8);
[agent1_gradient_x,agent1_gradient_y]=Calculate_gradient_dynamic(x1,x2,A1,F,agent1_x1,agent1_x2,10);
[agent2_gradient_x,agent2_gradient_y]=Calculate_gradient_dynamic(x1,x2,A1,F,agent2_x1,agent2_x2,10);
[agent4_gradient_x,agent4_gradient_y]=Calculate_gradient_dynamic(x1,x2,A1,F,agent4_x1,agent4_x2,10);
[agent5_gradient_x,agent5_gradient_y]=Calculate_gradient_dynamic(x1,x2,A1,F,agent5_x1,agent5_x2,10);
if sqrt( (x1-agent1_x1)^2+(x2-agent1_x2)^2 )<=30 %agent3 & agent1
    gradient_x=gradient_x+agent1_gradient_x;
    gradient_y=gradient_y+agent1_gradient_y;
end
if sqrt( (x1-agent2_x1)^2+(x2-agent2_x2)^2 )<=30 %agent3 & agent2
    gradient_x=gradient_x+agent2_gradient_x;
    gradient_y=gradient_y+agent2_gradient_y;
end
if sqrt( (x1-agent4_x1)^2+(x2-agent4_x2)^2 )<=30 %agent3 & agent4
    gradient_x=gradient_x+agent4_gradient_x;
    gradient_y=gradient_y+agent4_gradient_y;
end
if sqrt( (x1-agent5_x1)^2+(x2-agent5_x2)^2 )<=30 %agent3 & agent5
    gradient_x=gradient_x+agent5_gradient_x;
    gradient_y=gradient_y+agent5_gradient_y;
end
gradient_x=gradient_x;
gradient_y=gradient_y;
gradient_z=0;

Gradient_all=[gradient_x;gradient_y;gradient_z];
Li=0.2;
Bi=[0,cos(pi/6),-cos(pi/6);
    -1,sin(pi/6),sin(pi/6);
    Li,Li,Li;];

R1=[cos(xa3),-sin(xa3),0;
    sin(xa3),cos(xa3),0;
    0,0,1;];
R=0.02;
gx=R1*inv(Bi')*R;
A=Gradient_all'*gx;

%H=[1];
%H=[1,0;0,1];
%H=[0,0,0;0,0,0;0,0,0];
% H=[1,0,0;0,1,0;0,0,1];
 H=(1/2)*gx'*gx;
b=[0];
F=[-2*gx'*40*Gradient_all];
%=[];
u1=0;u2=0;u3=0;
U=PVF_optimizer(H,b,A,F,distance,gradient_x,gradient_y);

u1=U(1,1);
u2=U(2,1);
u3=U(3,1);

== matlab function scenario_2_TAC_5robots_plus_2019/agent3/STL_barrier 1 ==
  data: b output; b50 output; b1 output; b2 output; yita output; h output; t input; p1 input; p2 input; L1 input; L2 input; yita50 output; h50 output; agent1_x1 input; agent1_x2 input; agent2_x1 input; agent2_x2 input; agent4_x1 input; agent4_x2 input; agent5_x1 input; agent5_x2 input
function [b,b50,b1,b2,yita,h,yita50,h50] = fcn(t,p1,p2,L1,L2,agent1_x1,agent1_x2,agent2_x1,agent2_x2,agent4_x1,agent4_x2,agent5_x1,agent5_x2 )
d1=L1;
d2=L2;

d11=-50;
d22=0;

d111=0;d222=30;

b=25*exp(-0.32*t)+5-sqrt( (p1-d1)^2 + (p2-d2)^2 ); %STL_tracking
yita=-25*exp(-0.32*t)+10;
h=15-sqrt( (p1-d1)^2 + (p2-d2)^2 );


b50=60*exp(-0.125*(t))+5-sqrt( (p1-d11)^2 + (p2-d22)^2 );%STL_visiting 
yita50=-60*exp(-0.125*(t))+5;
h50=10-sqrt( (p1-d11)^2 + (p2-d22)^2 );


% b50=5-sqrt( (p1-d11)^2 + (p2-d22)^2 );
% yita50=5;
% h50=10-sqrt( (p1-d11)^2 + (p2-d22)^2 );

b1=sqrt( (p1-d11)^2 + (p2-d22)^2 )-0;%STL_visiting_trigger

b21=sqrt( (p1-d111)^2 + (p2-d222)^2 )-6;
b3_1=sqrt( (p1-agent1_x1)^2 + (p2-agent1_x2)^2 )-10;
b3_2=sqrt( (p1-agent2_x1)^2 + (p2-agent2_x2)^2 )-10;
b3_4=sqrt( (p1-agent4_x1)^2 + (p2-agent4_x2)^2 )-10;
b3_5=sqrt( (p1-agent5_x1)^2 + (p2-agent5_x2)^2 )-10;
b2=-(1/20)*log(exp(-20*b21)+exp(-20*b3_1)+exp(-20*b3_2)+exp(-20*b3_4)+exp(-20*b3_5)); %obstacle_avoidence_trigger

== matlab function scenario_2_TAC_5robots_plus_2019/agent3/STL_controller1_visiting ==
  data: x1 input; x2 input; L1 input; L2 input; b_in input; u1 output; xa3 input; u2 output; u3 output; t input
function [u1,u2,u3]= fcn(x1, x2,L1,L2, b_in, xa3,t)
coder.extrinsic('quadoptimizer');
%coder.extrinsic('save');
d1=-50; d2=0;

partial_b=(1/2)*((x1-d1)^2+(x2-d2)^2)^(-1/2);
partial_b_x=[-2*partial_b*(x1-d1),-2*partial_b*(x2-d2),0];


Li=0.2;
Bi=[0,cos(pi/6),-cos(pi/6);
    -1,sin(pi/6),sin(pi/6);
    Li,Li,Li;];

R1=[cos(xa3),-sin(xa3),0;
    sin(xa3),cos(xa3),0;
    0,0,1;];
R=0.02;

gx=R1*inv(Bi')*R;

A=partial_b_x*gx;

H=[1,0,0;0,1,0;0,0,1];
%H=[1];

b=300*b_in-0.125*60*exp(-0.125*(t))-50;

%  b=500*b_in-50;


u1=0;u2=0;u3=0;
U=quadoptimizer(H,b,A);

%U=quadprod(H,[],-A,b);

u1=U(1,1);
u2=U(2,1);
u3=U(3,1);

== matlab function scenario_2_TAC_5robots_plus_2019/agent3/STL_controller_tracking1 ==
  data: x1 input; x2 input; L1 input; L2 input; b_in input; u1 output; xa3 input; u2 output; u3 output; t input
function [u1,u2,u3]= fcn(x1, x2,L1,L2, b_in, xa3,t)
coder.extrinsic('quadoptimizer');
%coder.extrinsic('save');
d1=L1; d2=L2;

partial_b=(1/2)*((x1-d1)^2+(x2-d2)^2)^(-1/2);
partial_b_x=[-2*partial_b*(x1-d1),-2*partial_b*(x2-d2),0];
partial_b_L=[2*partial_b*(x1-d1),2*partial_b*(x2-d2)];
pho1=sqrt(partial_b_L(1,1)^2+partial_b_L(1,2)^2);
Li=0.2;
Bi=[0,cos(pi/6),-cos(pi/6);
    -1,sin(pi/6),sin(pi/6);
    Li,Li,Li;];

R1=[cos(xa3),-sin(xa3),0;
    sin(xa3),cos(xa3),0;
    0,0,1;];
R=0.02;

gx=R1*inv(Bi')*R;

A=partial_b_x*gx;

H=[1,0,0;0,1,0;0,0,1];
%H=[1];

% b=200*b_in-0.37*25*exp(-0.37*t)-300-30*pho1;
b=200*b_in-0.32*25*exp(-0.32*t)-300-30*pho1;


u1=0;u2=0;u3=0;
U=quadoptimizer(H,b,A);

%U=quadprod(H,[],-A,b);

u1=U(1,1);
u2=U(2,1);
u3=U(3,1);

== matlab function scenario_2_TAC_5robots_plus_2019/agent3/leader1 ==
  data: t input; L1 output; L2 output
function [L1,L2] = fcn(t)
L1=-30*sin(1*t);
L2=-30*cos(1*t);

== matlab function scenario_2_TAC_5robots_plus_2019/agent3/omnidirectional robot1 ==
  data: ua1 input; xa1_dot output; ua2 input; ua3 input; xa3 input; xa2_dot output; xa3_dot output
function [xa1_dot,xa2_dot,xa3_dot]= fcn(ua1,ua2,ua3,xa3)

Li=0.2;
Bi=[0,cos(pi/6),-cos(pi/6);
    -1,sin(pi/6),sin(pi/6);
    Li,Li,Li;];

R1=[cos(xa3),-sin(xa3),0;
    sin(xa3),cos(xa3),0;
    0,0,1;];
R=0.02;

A=R1*inv(Bi')*R*[ua1;ua2;ua3];
xa1_dot=A(1,1);
xa2_dot=A(2,1);
xa3_dot=A(3,1);

== matlab function scenario_2_TAC_5robots_plus_2019/agent3/regulation function  ==
  data: STL_u1 input; U1 output; STL_u2 input; STL_u3 input; STLv_u1 input; STLv_u2 input; STLv_u3 input; obs_u1 input; obs_u2 input; obs_u3 input; b1 input; U2 output; U3 output; b2 input
function [U1,U2,U3] = fcn(STL_u1,STL_u2,STL_u3,STLv_u1,STLv_u2,STLv_u3,obs_u1,obs_u2,obs_u3,b1,b2)
U_track=[STL_u1;STL_u2;STL_u3];
U_visit=[STLv_u1;STLv_u2;STLv_u3];
U_obs=[obs_u1;obs_u2;obs_u3];

k=0.065;
lambda=1-exp(-k*max(b1,0));
U_goal=lambda*U_track+(1-lambda)*U_visit;
% U_goal=[0;0;0];
% U_goal=U_track;
j=0.15;
gamma=1-exp(-j*max(b2,0));
U=gamma*U_goal+(1-gamma)*U_obs;

% U=U_goal;
U1=0;U2=0;U3=0;
U1=U(1,1);
U2=U(2,1);
U3=U(3,1);

== matlab function scenario_2_TAC_5robots_plus_2019/agent3/velocity_constraint1 ==
  data: U1 input; Uc1 output; U2 input; U3 input; xa3 input; v_max input; Uc2 output; Uc3 output
function [Uc1,Uc2,Uc3] = fcn(U1,U2,U3,xa3,v_max)

Li=0.2;
Bi=[0,cos(pi/6),-cos(pi/6);
    -1,sin(pi/6),sin(pi/6);
    Li,Li,Li;];

R1=[cos(xa3),-sin(xa3),0;
    sin(xa3),cos(xa3),0;
    0,0,1;];
R=0.02;
gx=R1*inv(Bi')*R;

U=[U1;U2;U3];
V=[0;0;0];
V=gx*U;
if V(1,1)^2+V(2,1)^2<=v_max^2
     U(1,1)= U(1,1);
     U(2,1)= U(2,1);
else 
    U(1,1)=sqrt(v_max^2/(V(1,1)^2+V(2,1)^2))*U(1,1);
    U(2,1)=sqrt(v_max^2/(V(1,1)^2+V(2,1)^2))*U(2,1);
    U(3,1)=sqrt(v_max^2/(V(1,1)^2+V(2,1)^2))*U(3,1);
end

Uc1=U(1,1);
Uc2=U(2,1);
Uc3=U(3,1);

== matlab function scenario_2_TAC_5robots_plus_2019/distance ==
  data: agent1_x1 input; distance_1_2 output; agent1_x2 input; agent2_x1 input; agent2_x2 input; agent3_x1 input; agent3_x2 input; agent4_x1 input; agent4_x2 input; agent5_x1 input; agent5_x2 input; distance_1_3 output; distance_1_4 output; distance_1_5 output; distance_2_3 output; distance_2_4 output; distance_2_5 output; distance_3_4 output; distance_3_5 output; distance_4_5 output
function [distance_1_2,distance_1_3,distance_1_4,distance_1_5,distance_2_3,distance_2_4,distance_2_5,distance_3_4,distance_3_5,distance_4_5]  = fcn(agent1_x1,agent1_x2,agent2_x1,agent2_x2,agent3_x1,agent3_x2,agent4_x1,agent4_x2,agent5_x1,agent5_x2)
distance_1_2=sqrt( (agent1_x1-agent2_x1)^2+ (agent1_x2-agent2_x2 )^2  );
distance_1_3=sqrt( (agent1_x1-agent3_x1)^2+ (agent1_x2-agent3_x2 )^2  );
distance_1_4=sqrt( (agent1_x1-agent4_x1)^2+ (agent1_x2-agent4_x2 )^2  );
distance_1_5=sqrt( (agent1_x1-agent5_x1)^2+ (agent1_x2-agent5_x2 )^2  );
distance_2_3=sqrt( (agent2_x1-agent3_x1)^2+ (agent2_x2-agent3_x2 )^2  );
distance_2_4=sqrt( (agent2_x1-agent4_x1)^2+ (agent2_x2-agent4_x2 )^2  );
distance_2_5=sqrt( (agent2_x1-agent5_x1)^2+ (agent2_x2-agent5_x2 )^2  );
distance_3_4=sqrt( (agent3_x1-agent4_x1)^2+ (agent3_x2-agent4_x2 )^2  );
distance_3_5=sqrt( (agent3_x1-agent5_x1)^2+ (agent3_x2-agent5_x2 )^2  );
distance_4_5=sqrt( (agent4_x1-agent5_x1)^2+ (agent4_x2-agent5_x2 )^2  );

== matlab function scenario_2_TAC_5robots_plus_2019/agent4/MATLAB Function2 ==
  data: x1 input; theta output; y1 input
function theta = fcn(x1, y1)
theta=atan2(y1,x1);

== matlab function scenario_2_TAC_5robots_plus_2019/agent4/Potential_Field_controller3 ==
  data: x1 input; x2 input; agent1_x1 input; agent1_x2 input; agent2_x1 input; agent2_x2 input; agent3_x1 input; agent3_x2 input; agent5_x1 input; agent5_x2 input; L1 input; L2 input; u1 output; xa3 input; u2 output; u3 output
function [u1,u2,u3] = fcn(x1, x2, agent1_x1,agent1_x2,agent2_x1,agent2_x2,agent3_x1,agent3_x2,agent5_x1,agent5_x2,L1,L2, xa3)
coder.extrinsic('Calculate_gradient');
coder.extrinsic('Calculate_gradient_x15');
coder.extrinsic('PVF_optimizer');
coder.extrinsic('add_random');
A1=[-1,0;0,-1];
F=[2*L1,2*L2];
distance=sqrt((x1-90)^2+(x2-90)^2);

gradient_x=0;gradient_y=0;
agent1_gradient_x=0;agent1_gradient_y=0;
agent2_gradient_x=0;agent2_gradient_y=0;
agent3_gradient_x=0;agent3_gradient_y=0;
agent5_gradient_x=0;agent5_gradient_y=0;
[gradient_x,gradient_y]=Calculate_gradient(x1,x2,A1,F,0,30,8);
[agent1_gradient_x,agent1_gradient_y]=Calculate_gradient_dynamic(x1,x2,A1,F,agent1_x1,agent1_x2,10);
[agent2_gradient_x,agent2_gradient_y]=Calculate_gradient_dynamic(x1,x2,A1,F,agent2_x1,agent2_x2,10);
[agent3_gradient_x,agent3_gradient_y]=Calculate_gradient_dynamic(x1,x2,A1,F,agent3_x1,agent3_x2,10);
[agent5_gradient_x,agent5_gradient_y]=Calculate_gradient_dynamic(x1,x2,A1,F,agent5_x1,agent5_x2,10);
if sqrt( (x1-agent1_x1)^2+(x2-agent1_x2)^2 )<=30 %agent4 & agent1
    gradient_x=gradient_x+agent1_gradient_x;
    gradient_y=gradient_y+agent1_gradient_y;
end
if sqrt( (x1-agent2_x1)^2+(x2-agent2_x2)^2 )<=30 %agent4 & agent2
    gradient_x=gradient_x+agent2_gradient_x;
    gradient_y=gradient_y+agent2_gradient_y;
end
if sqrt( (x1-agent3_x1)^2+(x2-agent3_x2)^2 )<=30 %agent4 & agent3
    gradient_x=gradient_x+agent3_gradient_x;
    gradient_y=gradient_y+agent3_gradient_y;
end
if sqrt( (x1-agent5_x1)^2+(x2-agent5_x2)^2 )<=30 %agent4 & agent5
    gradient_x=gradient_x+agent5_gradient_x;
    gradient_y=gradient_y+agent5_gradient_y;
end
gradient_x=gradient_x;
gradient_y=gradient_y;
gradient_z=0;

Gradient_all=[gradient_x;gradient_y;gradient_z];
Li=0.2;
Bi=[0,cos(pi/6),-cos(pi/6);
    -1,sin(pi/6),sin(pi/6);
    Li,Li,Li;];

R1=[cos(xa3),-sin(xa3),0;
    sin(xa3),cos(xa3),0;
    0,0,1;];
R=0.02;
gx=R1*inv(Bi')*R;
A=Gradient_all'*gx;

%H=[1];
%H=[1,0;0,1];
%H=[0,0,0;0,0,0;0,0,0];
% H=[1,0,0;0,1,0;0,0,1];
 H=(1/2)*gx'*gx;
b=[0];
F=[-2*gx'*40*Gradient_all];
%=[];
u1=0;u2=0;u3=0;
U=PVF_optimizer(H,b,A,F,distance,gradient_x,gradient_y);

u1=U(1,1);
u2=U(2,1);
u3=U(3,1);

== matlab function scenario_2_TAC_5robots_plus_2019/agent2/MATLAB Function2 ==
  data: x1 input; theta output; y1 input
function theta = fcn(x1, y1)
theta=atan2(y1,x1);

== matlab function scenario_2_TAC_5robots_plus_2019/agent4/STL_barrier 1 ==
  data: b output; b50 output; b1 output; b2 output; yita output; h output; t input; p1 input; p2 input; L1 input; L2 input; yita50 output; h50 output; agent1_x1 input; agent1_x2 input; agent2_x1 input; agent2_x2 input; agent3_x1 input; agent3_x2 input; agent5_x1 input; agent5_x2 input
function [b,b50,b1,b2,yita,h,yita50,h50] = fcn(t,p1,p2,L1,L2, agent1_x1,agent1_x2,agent2_x1,agent2_x2,agent3_x1,agent3_x2,agent5_x1,agent5_x2)
d1=L1;
d2=L2;

d11=-50;
d22=0;

d111=0;d222=30;

b=25*exp(-0.32*t)+5-sqrt( (p1-d1)^2 + (p2-d2)^2 ); %STL_tracking
yita=-25*exp(-0.32*t)+10;
h=15-sqrt( (p1-d1)^2 + (p2-d2)^2 );


b50=60*exp(-0.125*(t))+5-sqrt( (p1-d11)^2 + (p2-d22)^2 );%STL_visiting 
yita50=-60*exp(-0.125*(t))+5;
h50=10-sqrt( (p1-d11)^2 + (p2-d22)^2 );


% b50=5-sqrt( (p1-d11)^2 + (p2-d22)^2 );
% yita50=5;
% h50=10-sqrt( (p1-d11)^2 + (p2-d22)^2 );

b1=sqrt( (p1-d11)^2 + (p2-d22)^2 )-0;%STL_visiting_trigger

b21=sqrt( (p1-d111)^2 + (p2-d222)^2 )-6;
b4_1=sqrt( (p1-agent1_x1)^2 + (p2-agent1_x2)^2 )-10;
b4_2=sqrt( (p1-agent2_x1)^2 + (p2-agent2_x2)^2 )-10;
b4_3=sqrt( (p1-agent3_x1)^2 + (p2-agent3_x2)^2 )-10;
b4_5=sqrt( (p1-agent5_x1)^2 + (p2-agent5_x2)^2 )-10;
% b22=sqrt( (p1-agent5_x1)^2 + (p2-agent5_x2)^2 )-6;
b2=-(1/20)*log(exp(-20*b21)+exp(-20*b4_1)+exp(-20*b4_2)+exp(-20*b4_3)+exp(-20*b4_5)); %obstacle_avoidence_trigger

== matlab function scenario_2_TAC_5robots_plus_2019/agent4/STL_controller1_visiting ==
  data: x1 input; x2 input; L1 input; L2 input; b_in input; u1 output; xa3 input; u2 output; u3 output; t input
function [u1,u2,u3]= fcn(x1, x2,L1,L2, b_in, xa3,t)
coder.extrinsic('quadoptimizer');
%coder.extrinsic('save');
d1=-50; d2=0;

partial_b=(1/2)*((x1-d1)^2+(x2-d2)^2)^(-1/2);
partial_b_x=[-2*partial_b*(x1-d1),-2*partial_b*(x2-d2),0];


Li=0.2;
Bi=[0,cos(pi/6),-cos(pi/6);
    -1,sin(pi/6),sin(pi/6);
    Li,Li,Li;];

R1=[cos(xa3),-sin(xa3),0;
    sin(xa3),cos(xa3),0;
    0,0,1;];
R=0.02;

gx=R1*inv(Bi')*R;

A=partial_b_x*gx;

H=[1,0,0;0,1,0;0,0,1];
%H=[1];

b=300*b_in-0.125*60*exp(-0.125*(t))-50;

%  b=500*b_in-50;


u1=0;u2=0;u3=0;
U=quadoptimizer(H,b,A);

%U=quadprod(H,[],-A,b);

u1=U(1,1);
u2=U(2,1);
u3=U(3,1);

== matlab function scenario_2_TAC_5robots_plus_2019/agent4/STL_controller_tracking1 ==
  data: x1 input; x2 input; L1 input; L2 input; b_in input; u1 output; xa3 input; u2 output; u3 output; t input
function [u1,u2,u3]= fcn(x1, x2,L1,L2, b_in, xa3,t)
coder.extrinsic('quadoptimizer');
%coder.extrinsic('save');
d1=L1; d2=L2;

partial_b=(1/2)*((x1-d1)^2+(x2-d2)^2)^(-1/2);
partial_b_x=[-2*partial_b*(x1-d1),-2*partial_b*(x2-d2),0];
partial_b_L=[2*partial_b*(x1-d1),2*partial_b*(x2-d2)];
pho1=sqrt(partial_b_L(1,1)^2+partial_b_L(1,2)^2);
Li=0.2;
Bi=[0,cos(pi/6),-cos(pi/6);
    -1,sin(pi/6),sin(pi/6);
    Li,Li,Li;];

R1=[cos(xa3),-sin(xa3),0;
    sin(xa3),cos(xa3),0;
    0,0,1;];
R=0.02;

gx=R1*inv(Bi')*R;

A=partial_b_x*gx;

H=[1,0,0;0,1,0;0,0,1];
%H=[1];

% b=200*b_in-0.37*25*exp(-0.37*t)-300-30*pho1;
b=200*b_in-0.32*25*exp(-0.32*t)-300-30*pho1;


u1=0;u2=0;u3=0;
U=quadoptimizer(H,b,A);

%U=quadprod(H,[],-A,b);

u1=U(1,1);
u2=U(2,1);
u3=U(3,1);

== matlab function scenario_2_TAC_5robots_plus_2019/agent4/leader1 ==
  data: t input; L1 output; L2 output
function [L1,L2] = fcn(t)
L1=-30*cos(1*t);
L2=30*sin(1*t);

== matlab function scenario_2_TAC_5robots_plus_2019/agent4/omnidirectional robot1 ==
  data: ua1 input; xa1_dot output; ua2 input; ua3 input; xa3 input; xa2_dot output; xa3_dot output
function [xa1_dot,xa2_dot,xa3_dot]= fcn(ua1,ua2,ua3,xa3)

Li=0.2;
Bi=[0,cos(pi/6),-cos(pi/6);
    -1,sin(pi/6),sin(pi/6);
    Li,Li,Li;];

R1=[cos(xa3),-sin(xa3),0;
    sin(xa3),cos(xa3),0;
    0,0,1;];
R=0.02;

A=R1*inv(Bi')*R*[ua1;ua2;ua3];
xa1_dot=A(1,1);
xa2_dot=A(2,1);
xa3_dot=A(3,1);

== matlab function scenario_2_TAC_5robots_plus_2019/agent2/Potential_Field_controller3 ==
  data: x1 input; x2 input; agent1_x1 input; agent1_x2 input; agent3_x1 input; agent3_x2 input; agent4_x1 input; agent4_x2 input; agent5_x1 input; agent5_x2 input; L1 input; L2 input; u1 output; xa3 input; u2 output; u3 output
function [u1,u2,u3] = fcn(x1, x2,agent1_x1,agent1_x2,agent3_x1,agent3_x2,agent4_x1,agent4_x2,agent5_x1,agent5_x2,L1,L2, xa3)
coder.extrinsic('Calculate_gradient');
coder.extrinsic('Calculate_gradient_x15');
coder.extrinsic('PVF_optimizer');
coder.extrinsic('add_random');
A1=[-1,0;0,-1];
F=[2*L1,2*L2];
distance=sqrt((x1-90)^2+(x2-90)^2);

gradient_x=0;gradient_y=0;
agent1_gradient_x=0;agent1_gradient_y=0;
agent3_gradient_x=0;agent3_gradient_y=0;
agent4_gradient_x=0;agent4_gradient_y=0;
agent5_gradient_x=0;agent5_gradient_y=0;
[gradient_x,gradient_y]=Calculate_gradient(x1,x2,A1,F,0,30,8);
[agent1_gradient_x,agent1_gradient_y]=Calculate_gradient_dynamic(x1,x2,A1,F,agent1_x1,agent1_x2,10);
[agent3_gradient_x,agent3_gradient_y]=Calculate_gradient_dynamic(x1,x2,A1,F,agent3_x1,agent3_x2,10);
[agent4_gradient_x,agent4_gradient_y]=Calculate_gradient_dynamic(x1,x2,A1,F,agent4_x1,agent4_x2,10);
[agent5_gradient_x,agent5_gradient_y]=Calculate_gradient_dynamic(x1,x2,A1,F,agent5_x1,agent5_x2,10);
if sqrt( (x1-agent1_x1)^2+(x2-agent1_x2)^2 )<=30 %agent2 & agent1
    gradient_x=gradient_x+agent1_gradient_x;
    gradient_y=gradient_y+agent1_gradient_y;
end
if sqrt( (x1-agent3_x1)^2+(x2-agent3_x2)^2 )<=30 %agent2 & agent3
    gradient_x=gradient_x+agent3_gradient_x;
    gradient_y=gradient_y+agent3_gradient_y;
end
if sqrt( (x1-agent4_x1)^2+(x2-agent4_x2)^2 )<=30 %agent2 & agent4
    gradient_x=gradient_x+agent4_gradient_x;
    gradient_y=gradient_y+agent4_gradient_y;
end
if sqrt( (x1-agent5_x1)^2+(x2-agent5_x2)^2 )<=30 %agent2 & agent5
    gradient_x=gradient_x+agent5_gradient_x;
    gradient_y=gradient_y+agent5_gradient_y;
end
gradient_x=gradient_x;
gradient_y=gradient_y;
gradient_z=0;

Gradient_all=[gradient_x;gradient_y;gradient_z];
Li=0.2;
Bi=[0,cos(pi/6),-cos(pi/6);
    -1,sin(pi/6),sin(pi/6);
    Li,Li,Li;];

R1=[cos(xa3),-sin(xa3),0;
    sin(xa3),cos(xa3),0;
    0,0,1;];
R=0.02;
gx=R1*inv(Bi')*R;
A=Gradient_all'*gx;

%H=[1];
%H=[1,0;0,1];
%H=[0,0,0;0,0,0;0,0,0];
% H=[1,0,0;0,1,0;0,0,1];
 H=(1/2)*gx'*gx;
b=[0];
F=[-2*gx'*40*Gradient_all];
%=[];
u1=0;u2=0;u3=0;
U=PVF_optimizer(H,b,A,F,distance,gradient_x,gradient_y);

u1=U(1,1);
u2=U(2,1);
u3=U(3,1);

== matlab function scenario_2_TAC_5robots_plus_2019/agent4/regulation function  ==
  data: STL_u1 input; U1 output; STL_u2 input; STL_u3 input; STLv_u1 input; STLv_u2 input; STLv_u3 input; obs_u1 input; obs_u2 input; obs_u3 input; b1 input; U2 output; U3 output; b2 input
function [U1,U2,U3] = fcn(STL_u1,STL_u2,STL_u3,STLv_u1,STLv_u2,STLv_u3,obs_u1,obs_u2,obs_u3,b1,b2)
U_track=[STL_u1;STL_u2;STL_u3];
U_visit=[STLv_u1;STLv_u2;STLv_u3];
U_obs=[obs_u1;obs_u2;obs_u3];

k=0.065;
lambda=1-exp(-k*max(b1,0));
U_goal=lambda*U_track+(1-lambda)*U_visit;
% U_goal=[0;0;0];
% U_goal=U_track;
j=0.15;
gamma=1-exp(-j*max(b2,0));
U=gamma*U_goal+(1-gamma)*U_obs;

% U=U_goal;
U1=0;U2=0;U3=0;
U1=U(1,1);
U2=U(2,1);
U3=U(3,1);

== matlab function scenario_2_TAC_5robots_plus_2019/agent4/velocity_constraint1 ==
  data: U1 input; Uc1 output; U2 input; U3 input; xa3 input; v_max input; Uc2 output; Uc3 output
function [Uc1,Uc2,Uc3] = fcn(U1,U2,U3,xa3,v_max)

Li=0.2;
Bi=[0,cos(pi/6),-cos(pi/6);
    -1,sin(pi/6),sin(pi/6);
    Li,Li,Li;];

R1=[cos(xa3),-sin(xa3),0;
    sin(xa3),cos(xa3),0;
    0,0,1;];
R=0.02;
gx=R1*inv(Bi')*R;

U=[U1;U2;U3];
V=[0;0;0];
V=gx*U;
if V(1,1)^2+V(2,1)^2<=v_max^2
     U(1,1)= U(1,1);
     U(2,1)= U(2,1);
else 
    U(1,1)=sqrt(v_max^2/(V(1,1)^2+V(2,1)^2))*U(1,1);
    U(2,1)=sqrt(v_max^2/(V(1,1)^2+V(2,1)^2))*U(2,1);
    U(3,1)=sqrt(v_max^2/(V(1,1)^2+V(2,1)^2))*U(3,1);
end

Uc1=U(1,1);
Uc2=U(2,1);
Uc3=U(3,1);

== matlab function scenario_2_TAC_5robots_plus_2019/agent5/MATLAB Function2 ==
  data: x1 input; theta output; y1 input
function theta = fcn(x1, y1)
theta=atan2(y1,x1);
